simulink model "D_P_I_O"  (R2016b)
settings: Solver=ode45  StartTime=0.0  StopTime=TSIM  RelTol=1e-3  EnableMultiTasking=on
values from neighbouring files (symbols this model uses):
  ALPC = A-LP*c1    [D_PIO.m]    (also in D_PIO_Robust.m)
  c1 = [0 1 0 0 0 0 0 ... (first row only)    [DPIO.m]    (also in D_PIO.m; D_PIO_Robust.m)
  ddot0 = 0    [D_PIO.m]    (also in D_PIO_Robust.m)
  Ed = d2    [DPIO.m]    (also in D_PIO.m = [d2,zeros(7,1) ,zeros(7,1)]; D_PIO_Robust.m = [d2,zeros(7,1) ,zeros(7,1)])
  f1Val = 10    [DPIO.m]    (also in D_PIO.m; D_PIO_Robust.m)
  f2Val = 10    [DPIO.m]    (also in D_PIO.m; D_PIO_Robust.m)
  f3Val = 10    [DPIO.m]    (also in D_PIO.m; D_PIO_Robust.m)
  f4Val = 10    [DPIO.m]    (also in D_PIO.m; D_PIO_Robust.m)
  f5Val = 10    [DPIO.m]    (also in D_PIO.m; D_PIO_Robust.m)
  f6Val = 10    [DPIO.m]    (also in D_PIO.m; D_PIO_Robust.m)
  f7Val = 10    [DPIO.m]    (also in D_PIO.m; D_PIO_Robust.m)
  flt1 = 0    [DPIO.m]    (also in D_PIO.m; D_PIO_Robust.m)
  flt2 = 1    [DPIO.m]    (also in D_PIO.m; D_PIO_Robust.m)
  flt3 = 0    [DPIO.m]    (also in D_PIO.m; D_PIO_Robust.m)
  flt4 = 0    [DPIO.m]    (also in D_PIO.m; D_PIO_Robust.m)
  flt5 = 0    [DPIO.m]    (also in D_PIO.m; D_PIO_Robust.m)
  flt6 = 0    [DPIO.m]    (also in D_PIO.m; D_PIO_Robust.m)
  flt7 = 0    [DPIO.m]    (also in D_PIO.m; D_PIO_Robust.m)
  L = Deg-Ag    [DPIO.m]    (also in D_PIO.m; D_PIO_Robust.m)
  LI = 10    [D_PIO.m]    (also in D_PIO_Robust.m)
  LP = place(A,c1',[-1,-2,-3,-4,-5,-6,-7])'    [D_PIO.m]    (also in D_PIO_Robust.m = Al*pCD)
  tf1 = 2    [DPIO.m]    (also in D_PIO.m; D_PIO_Robust.m)
  tf2 = 2    [DPIO.m]    (also in D_PIO.m; D_PIO_Robust.m)
  tf3 = 2    [DPIO.m]    (also in D_PIO.m; D_PIO_Robust.m)
  tf4 = 2    [DPIO.m]    (also in D_PIO.m; D_PIO_Robust.m)
  tf5 = 2    [DPIO.m]    (also in D_PIO.m; D_PIO_Robust.m)
  tf6 = 5    [DPIO.m]    (also in D_PIO.m; D_PIO_Robust.m)
  tf7 = 7    [DPIO.m]    (also in D_PIO.m; D_PIO_Robust.m)
  x0 = [0 1 1 0 0 0 0]    [DPIO.m]    (also in D_PIO.m; D_PIO_Robust.m)
  xdot0 = zeros(7,1)'    [D_PIO.m]    (also in D_PIO_Robust.m)
settings Model: Creator=sqn4594  LastModifiedBy=samnazari
settings DataIOCC: LimitDataPoints=on  SaveFormat=Array
settings OptimizationCC: LifeSpan=inf
settings DebuggingCC: SolverPrmCheckMsg=warning  FcnCallInpInsideContextMsg=warning  AllowSymbolicDim=off  SFUnexpectedBacktrackingDiag=warning  SFNoUnconditionalDefaultTransitionDiag=warning  SFExecutionAtInitializationDiag=none
settings HardwareCC: ProdBitPerPointer=32  ProdBitPerSizeT=32  ProdBitPerPtrDiffT=32  ProdLargestAtomicFloat=None  ProdIntDivRoundTo=Undefined  ProdEndianess=Unspecified  ProdWordSize=32  ProdHWDeviceType=32-bit Generic
settings ModelReferenceCC: PropagateSignalLabelsOutOfModel=off
settings GRTTargetCC: TargetLangStandard=C89/C90 (ANSI)  GeneratePreprocessorConditionals=Disable all
settings ConfigComp: CovMetricSettings=dw  CovHtmlReporting=on  CovSaveCumulativeToWorkspaceVar=on  CovSaveSingleToWorkspaceVar=on  CovExternalEMLEnable=off

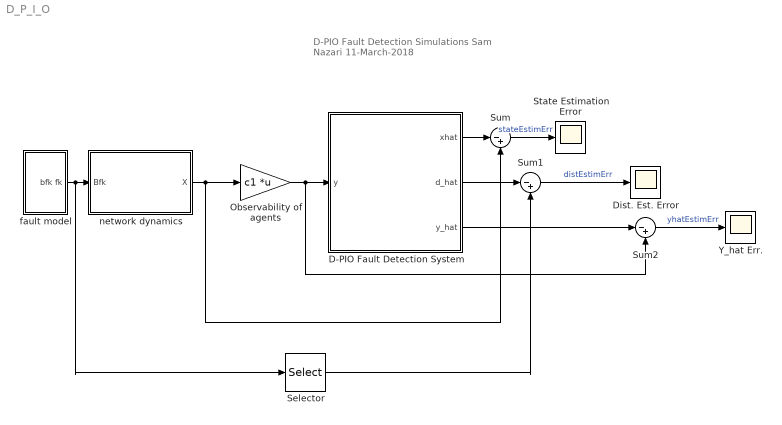
== system D_P_I_O ==
  note: D-PIO Fault Detection Simulations
      | Sam Nazari
      | 11-March-2018
  D-PIO Fault Detection System : Subsystem
  Dist. Est. Error : Scope
  "Observability of agents " : Gain  Gain=c1  Multiplication=Matrix(K*u)
  Selector : Selector  InputPortWidth=7  IndexOptions=Index vector (dialog)  Indices=[2 3 4]  OutputSizes=1
  State Estimation Error : Scope
  Sum : Sum  Inputs=|-+
  Sum1 : Sum  Inputs=|-+
  Sum2 : Sum  Inputs=|-+
  Y_hat Err. : Scope
  fault model : Subsystem
  network dynamics : Subsystem
  wires:
  fault model/1(bfk fk) -> Selector/1, network dynamics/1(Bfk)
  network dynamics/1(X) -> Sum/2, "Observability of agents "/1
  "Observability of agents "/1 -> Sum2/2, D-PIO Fault Detection System/1(y)
  D-PIO Fault Detection System/1("xhat ") -> Sum/1
  Sum/1 -> State Estimation Error/1  "stateEstimErr"
  D-PIO Fault Detection System/2("d_hat ") -> Sum1/1
  Selector/1 -> Sum1/2
  Sum1/1 -> Dist. Est. Error/1  "distEstimErr"
  D-PIO Fault Detection System/3("y_hat ") -> Sum2/1
  Sum2/1 -> Y_hat Err./1  "yhatEstimErr"

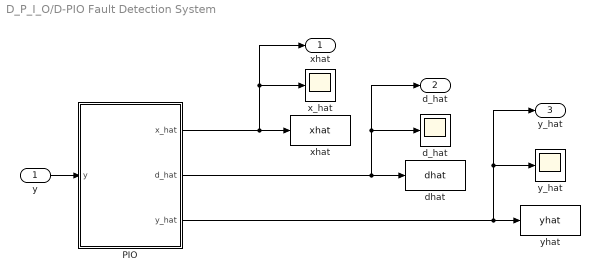
== system D_P_I_O/D-PIO Fault Detection System ==
  y : Inport
  PIO : Subsystem
  d_hat : Scope
  dhat : ToWorkspace  VariableName=dhat  SaveFormat=Timeseries  SampleTime=-1
  "x_hat " : Scope
  xhat : ToWorkspace  VariableName=xhat  SaveFormat=Timeseries  SampleTime=-1
  y_hat : Scope
  yhat : ToWorkspace  VariableName=yhat  SaveFormat=Timeseries  SampleTime=-1
  "xhat " : Outport
  "d_hat " : Outport  Port=2
  "y_hat " : Outport  Port=3
  wires:
  y/1 -> PIO/1(y)
  PIO/1(x_hat) -> "x_hat "/1, "xhat "/1, xhat/1
  PIO/2(d_hat) -> "d_hat "/1, d_hat/1, dhat/1
  PIO/3(y_hat) -> "y_hat "/1, y_hat/1, yhat/1

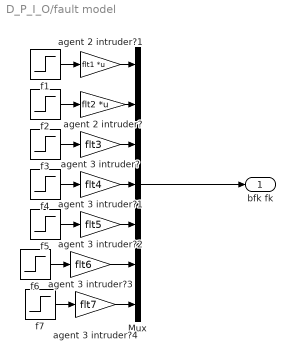
== system D_P_I_O/fault model ==
  Mux : Mux  Inputs=7
  agent 2 intruder? : Gain  Gain=flt2  Multiplication=Matrix(K*u)
  agent 2 intruder?1 : Gain  Gain=flt1  Multiplication=Matrix(K*u)
  agent 3 intruder? : Gain  Gain=flt3
  agent 3 intruder?1 : Gain  Gain=flt4
  agent 3 intruder?2 : Gain  Gain=flt5
  agent 3 intruder?3 : Gain  Gain=flt6
  agent 3 intruder?4 : Gain  Gain=flt7
  f1 : Step  After=f1Val  SampleTime=tf1
  f2 : Step  After=f2Val  SampleTime=tf2
  f3 : Step  After=f3Val  SampleTime=tf3
  f4 : Step  After=f4Val  SampleTime=tf4
  f5 : Step  After=f5Val  SampleTime=tf5
  f6 : Step  After=f6Val  SampleTime=tf6
  f7 : Step  After=f7Val  SampleTime=tf7
  bfk fk : Outport
  wires:
  Mux/1 -> bfk fk/1
  f1/1 -> agent 2 intruder?1/1
  f2/1 -> agent 2 intruder?/1
  f3/1 -> agent 3 intruder?/1
  agent 2 intruder?/1 -> Mux/2
  agent 3 intruder?/1 -> Mux/3
  agent 2 intruder?1/1 -> Mux/1
  f4/1 -> agent 3 intruder?1/1
  agent 3 intruder?1/1 -> Mux/4
  agent 3 intruder?2/1 -> Mux/5
  f5/1 -> agent 3 intruder?2/1
  f6/1 -> agent 3 intruder?3/1
  agent 3 intruder?3/1 -> Mux/6
  f7/1 -> agent 3 intruder?4/1
  agent 3 intruder?4/1 -> Mux/7

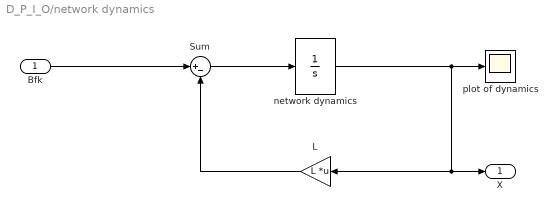
== system D_P_I_O/network dynamics ==
  Bfk : Inport
  L : Gain  Gain=L  Multiplication=Matrix(K*u)
  Sum : Sum  Inputs=|+-
  network dynamics : Integrator  InitialCondition=x0
  plot of dynamics : Scope
  X : Outport
  wires:
  Bfk/1 -> Sum/1
  Sum/1 -> network dynamics/1
  network dynamics/1 -> plot of dynamics/1, X/1, L/1
  L/1 -> Sum/2

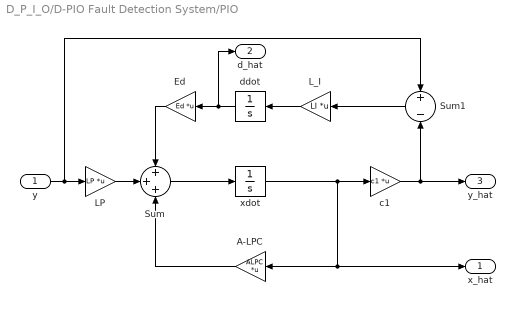
== system D_P_I_O/D-PIO Fault Detection System/PIO ==
  y : Inport
  A-LPC : Gain  Gain=ALPC  Multiplication=Matrix(K*u)
  Ed : Gain  Gain=Ed  Multiplication=Matrix(K*u)
  LP : Gain  Gain=LP  Multiplication=Matrix(K*u)
  L_I : Gain  Gain=LI  Multiplication=Matrix(K*u)
  Sum : Sum  Inputs=+++
  Sum1 : Sum  Inputs=+-
  c1 : Gain  Gain=c1  Multiplication=Matrix(K*u)
  ddot : Integrator  InitialCondition=ddot0
  xdot : Integrator  InitialCondition=xdot0
  x_hat : Outport
  d_hat : Outport  Port=2
  y_hat : Outport  Port=3
  wires:
  y/1 -> Sum1/1, LP/1
  A-LPC/1 -> Sum/3
  Sum/1 -> xdot/1
  L_I/1 -> ddot/1
  ddot/1 -> d_hat/1, Ed/1
  Ed/1 -> Sum/1
  LP/1 -> Sum/2
  xdot/1 -> x_hat/1, A-LPC/1, c1/1
  c1/1 -> y_hat/1, Sum1/2
  Sum1/1 -> L_I/1
